simulink model "pre_load_constant"  (R2021a)
settings: Solver=VariableStepAuto  StartTime=0.0  StopTime=10.0  RelTol=1e-3
PreLoadFcn:
  | K1=5;
  | K2=10;
settings Model: Creator=Acer  LastModifiedBy=Acer

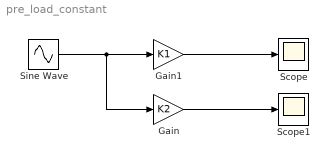
== system pre_load_constant ==
  Gain : Gain  Gain=K2
  Gain1 : Gain  Gain=K1
  Scope : Scope
  Scope1 : Scope
  Sine Wave : Sin  SampleTime=0
  wires:
  Sine Wave/1 -> Gain/1, Gain1/1
  Gain1/1 -> Scope/1
  Gain/1 -> Scope1/1
